simulink model "PSK"  (R2019a)
settings: Solver=VariableStepAuto  StartTime=0.0  StopTime=10.0  MaxStep=0.0001  RelTol=1e-3
libraries: commchan3 x1, dsparch4 x1, commrandsrc3 x1
settings Model: Creator=Lenovo  LastModifiedBy=MOSA

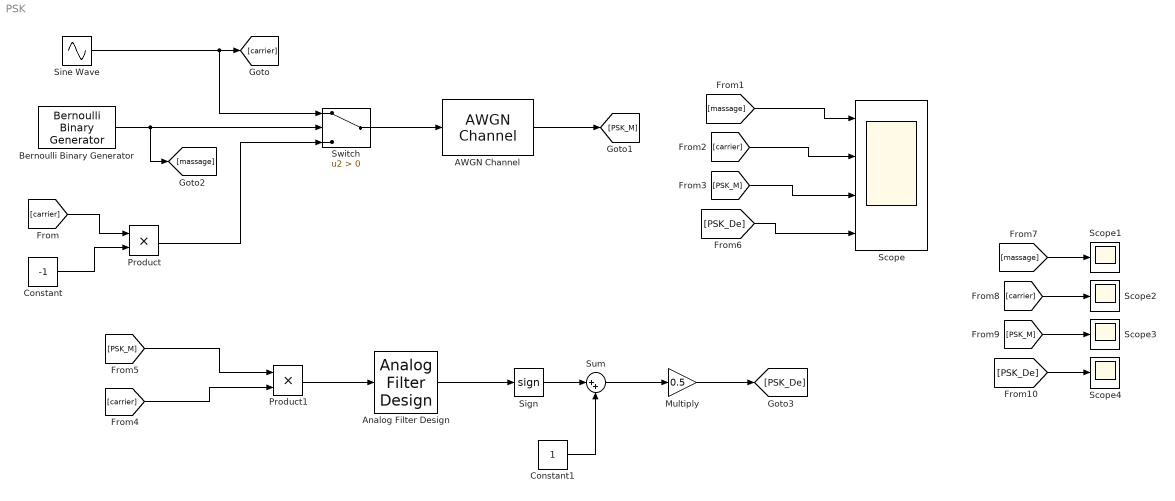
== system PSK ==
  AWGN Channel : commchan3/AWGN Channel  InputProcessing=Columns as channels (frame based)  seed=67  noiseMode="Signal to noise ratio  (SNR)"  EbNodB=10  EsNodB=10  SNRdB=10  bitsPerSym=1  Ps=1  Tsym=1  variance=1
  Analog Filter Design : dsparch4/Analog Filter Design  method=Butterworth  filttype=Lowpass  N=8  Wlo=35  Whi=35  Rp=2  Rs=40
  Bernoulli Binary Generator : commrandsrc3/Bernoulli Binary Generator  ProbabilityOfZero=0.5  SeedSource=Parameter  Seed=67  SampleTime=0.4  SamplesPerFrame=1  OutputDataType=double  SimulateUsing=Interpreted execution
  Constant : Constant  Value=-1
  Constant1 : Constant
  Multiply : Gain  Gain=0.5
  Product : Product
  Product1 : Product
  Scope : Scope  NumInputPorts=4
  Scope{1..4} (4 alike) : Scope
  Sign : Signum
  Sine Wave : Sin  Frequency=2*pi*5  SampleTime=0
  Sum : Sum  Inputs=|++
  Switch : Switch  Criteria=u2 > Threshold
  wires:
  Bernoulli Binary Generator/1 -> [massage], Switch/2
  Sine Wave/1 -> [carrier], Switch/1
  Product/1 -> Switch/3
  [carrier] -> Product/1
  Constant/1 -> Product/2
  [massage] -> Scope/1
  [carrier] -> Scope/2
  [PSK_M] -> Scope/3
  [carrier] -> Product1/2
  [PSK_M] -> Product1/1
  [PSK_De] -> Scope/4
  Switch/1 -> AWGN Channel/1
  Product1/1 -> Analog Filter Design/1
  AWGN Channel/1 -> [PSK_M]
  Analog Filter Design/1 -> Sign/1
  [massage] -> Scope1/1
  [carrier] -> Scope2/1
  [PSK_M] -> Scope3/1
  [PSK_De] -> Scope4/1
  Constant1/1 -> Sum/2
  Sign/1 -> Sum/1
  Sum/1 -> Multiply/1
  Multiply/1 -> [PSK_De]
